simulink library "stm32f4_rtc_lib"  (R2015b)
settings: Solver=ode45  StartTime=0.0  StopTime=10.0  RelTol=1e-3
libraries: simulink x46, amg_high_precision_rtc x5
settings Model: Creator=Krisada  LastModifiedBy=Aimagin
settings DataIOCC: SaveFormat=Array  SignalLoggingSaveFormat=ModelDataLogs
settings OptimizationCC: ExpressionDepthLimit=2147483647
settings DebuggingCC: UnderspecifiedInitializationDetection=Classic  MergeDetectMultiDrivingBlocksExec=none  SolverPrmCheckMsg=warning  FcnCallInpInsideContextMsg=UseLocalSettings  StateNameClashWarn=warning  StrictBusMsg=Warning
settings HardwareCC: ProdBitPerPointer=32  ProdLargestAtomicFloat=None  ProdIntDivRoundTo=Undefined  ProdEndianess=Unspecified  ProdWordSize=32  ProdHWDeviceType=32-bit Generic
settings GRTTargetCC: CombineOutputUpdateFcns=off  GRTInterface=on
settings ConfigComp: CovModelRefEnable=Off

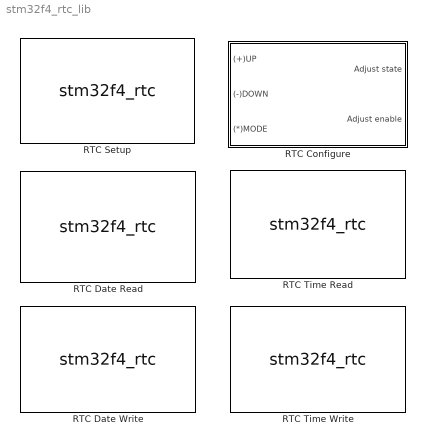
== system stm32f4_rtc_lib ==
  RTC Configure : Subsystem  mask{dummy=0}
      mask init:
      | stm32f4_rtc_configure_callback('init');
      mask Help: web(fullfile(waijungdocroot,'RTC_Configure.htm'), '-browser')
      mask Callback dummy: stm32f4_rtc_configure_callback('dummy');
      mask Display: text(0.5, 0.5, 'On-Chip RTC','ver','middle','hor','center');port_label('input', 1,'(+) UP');port_label('input', 2,'(-) DOWN');port_label('input', 3,'(*) MODE');port_label('output', 1,'State');port_label('output', 2,'Enable');
  RTC Date Read : S-Function  FunctionName=stm32f4_rtc  Parameters=inputtypearray,outputtypearray,confstr,sampletime,sampletimestr,blockid  SFunctionDeploymentMode=off  EnableBusSupport=off  mask(stm32f4_rtc){configuration=DateRead, clocksource=LSE (32.768kHz), dataformat=BIN, hourformat=HourFormat_24, inputtypearray=[0], outputtypearray=[4 3 3 3 3], confstr=["DateRead","LSE (32.768kHz)","BIN","HourFormat_24"], sampletime=-1, sampletimestr=0, blockid=stm32f4_rtc_libRTCDateRead}
      mask prompts: clocksource "Clock source"; dataformat "Format"; hourformat "Hour format"; inputtypearray "Input type array"; outputtypearray "Output type array"; confstr "Configuration string"; sampletime "Sample time (sec)"; sampletimestr "Compiled sample time (sec) in string"
      mask init:
      | stm32f4_rtc_callback('init');
      mask Help: web(fullfile(waijungdocroot,'stm32f4_rtc_read.htm'), '-browser')
      mask TypeOptions configuration: Setup | DateRead | TimeRead | DateWrite | TimeWrite
      mask Callback configuration: stm32f4_rtc_callback('configuration');
      mask TypeOptions clocksource: LSE (32.768kHz) | LSI
      mask TypeOptions dataformat: BCD | BIN
      mask Callback dataformat: stm32f4_rtc_callback('dataformat');
      mask TypeOptions hourformat: HourFormat_24 | HourFormat_12
      mask Callback confstr: stm32f4_rtc_callback('confstr');
      mask Callback sampletime: stm32f4_rtc_callback('sampletime');
      mask Callback sampletimestr: stm32f4_rtc_callback('sampletimestr');
      mask Callback blockid: stm32f4_rtc_callback('blockid');
      mask Display: text(0.05, 0.5, 'Module: RTC (DateRead)\nFormat: BIN\nTs (sec): 0','ver','middle','hor','left');port_label('output', 1,'Day');port_label('output', 2,'Date');port_label('output', 3,'Month');port_label('output', 4,'Year');
  RTC Date Write : S-Function  FunctionName=stm32f4_rtc  Parameters=inputtypearray,outputtypearray,confstr,sampletime,sampletimestr,blockid  SFunctionDeploymentMode=off  EnableBusSupport=off  mask(stm32f4_rtc){configuration=DateWrite, clocksource=LSE (32.768kHz), dataformat=BIN, hourformat=HourFormat_24, inputtypearray=[3 -1 -1 -1], outputtypearray=[0], confstr=["DateWrite","LSE (32.768kHz)","BIN","HourFormat_24"], sampletime=-1, sampletimestr=0, blockid=RTCDateWrite}
      mask prompts: clocksource "Clock source"; dataformat "Format"; hourformat "Hour format"; inputtypearray "Input type array"; outputtypearray "Output type array"; confstr "Configuration string"; sampletime "Sample time (sec)"; sampletimestr "Compiled sample time (sec) in string"
      mask init:
      | stm32f4_rtc_callback('init');
      mask Help: web(fullfile(waijungdocroot,'RTC_Date_Write.htm'), '-browser')
      mask TypeOptions configuration: Setup | DateRead | TimeRead | DateWrite | TimeWrite
      mask Callback configuration: stm32f4_rtc_callback('configuration');
      mask TypeOptions clocksource: LSE (32.768kHz) | LSI
      mask TypeOptions dataformat: BCD | BIN
      mask Callback dataformat: stm32f4_rtc_callback('dataformat');
      mask TypeOptions hourformat: HourFormat_24 | HourFormat_12
      mask Callback confstr: stm32f4_rtc_callback('confstr');
      mask Callback sampletime: stm32f4_rtc_callback('sampletime');
      mask Callback sampletimestr: stm32f4_rtc_callback('sampletimestr');
      mask Callback blockid: stm32f4_rtc_callback('blockid');
      mask Display: text(0.95, 0.5, 'Module: RTC (DateWrite)\nFormat: BIN\nTs (sec): 0','ver','middle','hor','right');port_label('input', 1,'Date');port_label('input', 2,'Month');port_label('input', 3,'Year');
  RTC Setup : S-Function  FunctionName=stm32f4_rtc  Parameters=inputtypearray,outputtypearray,confstr,sampletime,sampletimestr,blockid  SFunctionDeploymentMode=off  EnableBusSupport=off  mask(stm32f4_rtc){configuration=Setup, clocksource=LSI, dataformat=BIN, hourformat=HourFormat_24, inputtypearray=[0], outputtypearray=[0], confstr=["Setup","LSI","BIN","HourFormat_24"], sampletime=inf, sampletimestr=0, blockid=stm32f4_rtc_libRTCSetup}
      mask prompts: clocksource "Clock source"; dataformat "Format"; hourformat "Hour format"; inputtypearray "Input type array"; outputtypearray "Output type array"; confstr "Configuration string"; sampletime "Sample time (sec)"; sampletimestr "Compiled sample time (sec) in string"
      mask init:
      | stm32f4_rtc_callback('init');
      mask Help: web(fullfile(waijungdocroot,'stm32f4_rtc_setup.htm'), '-browser')
      mask TypeOptions configuration: Setup | DateRead | TimeRead | DateWrite | TimeWrite
      mask Callback configuration: stm32f4_rtc_callback('configuration');
      mask TypeOptions clocksource: LSE (32.768kHz) | LSI
      mask TypeOptions dataformat: BCD | BIN
      mask Callback dataformat: stm32f4_rtc_callback('dataformat');
      mask TypeOptions hourformat: HourFormat_24 | HourFormat_12
      mask Callback confstr: stm32f4_rtc_callback('confstr');
      mask Callback sampletime: stm32f4_rtc_callback('sampletime');
      mask Callback sampletimestr: stm32f4_rtc_callback('sampletimestr');
      mask Callback blockid: stm32f4_rtc_callback('blockid');
      mask Display: text(0.5, 0.5, 'Module: RTC (Setup)\nClock: LSI\nFormat: HourFormat_24\nTs (sec): 0','ver','middle','hor','center');
  RTC Time Read : S-Function  FunctionName=stm32f4_rtc  Parameters=inputtypearray,outputtypearray,confstr,sampletime,sampletimestr,blockid  SFunctionDeploymentMode=off  EnableBusSupport=off  mask(stm32f4_rtc){configuration=TimeRead, clocksource=LSE (32.768kHz), dataformat=BIN, hourformat=HourFormat_24, inputtypearray=[0], outputtypearray=[3 3 3 3], confstr=["TimeRead","LSE (32.768kHz)","BIN","HourFormat_24"], sampletime=-1, sampletimestr=0, blockid=stm32f4_rtc_libRTCTimeRead}
      mask prompts: clocksource "Clock source"; dataformat "Format"; hourformat "Hour format"; inputtypearray "Input type array"; outputtypearray "Output type array"; confstr "Configuration string"; sampletime "Sample time (sec)"; sampletimestr "Compiled sample time (sec) in string"
      mask init:
      | stm32f4_rtc_callback('init');
      mask Help: web(fullfile(waijungdocroot,'RTC_Time_Read.htm'), '-browser')
      mask TypeOptions configuration: Setup | DateRead | TimeRead | DateWrite | TimeWrite
      mask Callback configuration: stm32f4_rtc_callback('configuration');
      mask TypeOptions clocksource: LSE (32.768kHz) | LSI
      mask TypeOptions dataformat: BCD | BIN
      mask Callback dataformat: stm32f4_rtc_callback('dataformat');
      mask TypeOptions hourformat: HourFormat_24 | HourFormat_12
      mask Callback confstr: stm32f4_rtc_callback('confstr');
      mask Callback sampletime: stm32f4_rtc_callback('sampletime');
      mask Callback sampletimestr: stm32f4_rtc_callback('sampletimestr');
      mask Callback blockid: stm32f4_rtc_callback('blockid');
      mask Display: text(0.05, 0.5, 'Module: RTC (TimeRead)\nFormat: BIN\nTs (sec): 0','ver','middle','hor','left');port_label('output', 1,'Hour');port_label('output', 2,'Minute');port_label('output', 3,'Second');
  RTC Time Write : S-Function  FunctionName=stm32f4_rtc  Parameters=inputtypearray,outputtypearray,confstr,sampletime,sampletimestr,blockid  SFunctionDeploymentMode=off  EnableBusSupport=off  mask(stm32f4_rtc){configuration=TimeWrite, clocksource=LSE (32.768kHz), dataformat=BIN, hourformat=HourFormat_24, inputtypearray=[3 -1 -1 -1], outputtypearray=[0], confstr=["TimeWrite","LSE (32.768kHz)","BIN","HourFormat_24"], sampletime=-1, sampletimestr=0, blockid=stm32f4_rtc_libRTCTimeWrite}
      mask prompts: clocksource "Clock source"; dataformat "Format"; hourformat "Hour format"; inputtypearray "Input type array"; outputtypearray "Output type array"; confstr "Configuration string"; sampletime "Sample time (sec)"; sampletimestr "Compiled sample time (sec) in string"
      mask init:
      | stm32f4_rtc_callback('init');
      mask Help: web(fullfile(waijungdocroot,'RTC_Time_Write.htm'), '-browser')
      mask TypeOptions configuration: Setup | DateRead | TimeRead | DateWrite | TimeWrite
      mask Callback configuration: stm32f4_rtc_callback('configuration');
      mask TypeOptions clocksource: LSE (32.768kHz) | LSI
      mask TypeOptions dataformat: BCD | BIN
      mask Callback dataformat: stm32f4_rtc_callback('dataformat');
      mask TypeOptions hourformat: HourFormat_24 | HourFormat_12
      mask Callback confstr: stm32f4_rtc_callback('confstr');
      mask Callback sampletime: stm32f4_rtc_callback('sampletime');
      mask Callback sampletimestr: stm32f4_rtc_callback('sampletimestr');
      mask Callback blockid: stm32f4_rtc_callback('blockid');
      mask Display: text(0.95, 0.5, 'Module: RTC (TimeWrite)\nFormat: BIN\nTs (sec): 0','ver','middle','hor','right');port_label('input', 1,'Hour');port_label('input', 2,'Minute');port_label('input', 3,'Second');

== system stm32f4_rtc_lib/RTC Configure ==
  (+)UP : Inport
  (-)DOWN : Inport  Port=2
  (*)MODE : Inport  Port=3
  Debouce4 : Subsystem  TreatAsAtomicUnit=on  mask{mode=Toggle Latch, prescale=256, debouce=255}
      mask prompts: prescale "Prescale (Debouce count)"; debouce "Debouce value"
      settings: RTWFcnNameOpts=Use subsystem name  RTWFileNameOpts=Use function name
      mask TypeOptions mode: Normal | Single Pulse | Toggle Latch
      mask Callback mode: waijung_intput_validation_callback('mode');
      mask TypeOptions prescale: 4 | 8 | 16 | 32 | 64 | 128 | 256 | 512 | 1024 | 2048 | 4096 | 8192
      mask Callback debouce: waijung_intput_validation_callback('prescale');
      mask Display: disp('Button Pressed\n(Toggle Latch)\nDebouce count: 256');
  Enabled Subsystem : Subsystem  TreatAsAtomicUnit=on
  Adjust state : Outport
  Adjust enable : Outport  Port=2
  wires:
  (+)UP/1 -> Enabled Subsystem/1(UP)
  (-)DOWN/1 -> Enabled Subsystem/2(DOWN)
  (*)MODE/1 -> Debouce4/1(In1), Enabled Subsystem/3(MODE)
  Debouce4/1(Out1) -> Enabled Subsystem/Enable, Adjust enable/1
  Enabled Subsystem/1(Adjust state) -> Adjust state/1

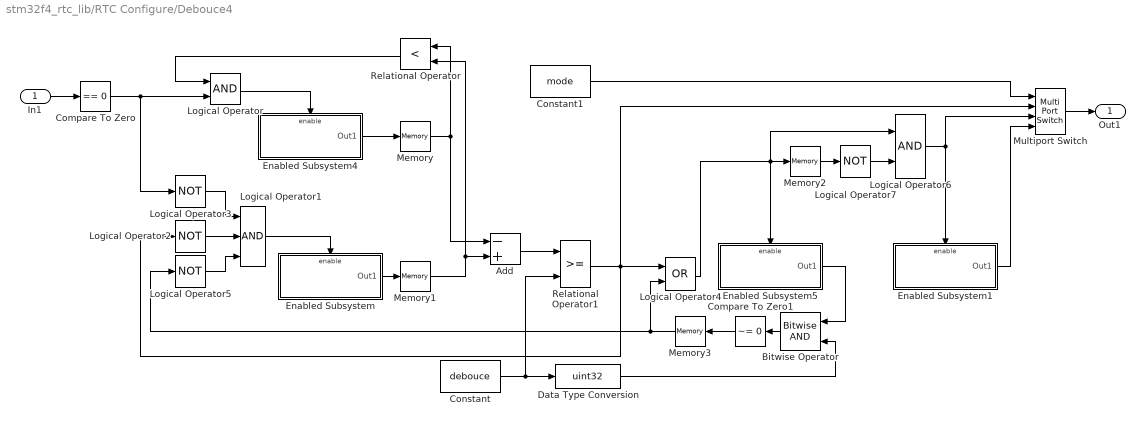
== system stm32f4_rtc_lib/RTC Configure/Debouce4 ==
  In1 : Inport
  Add : Sum  Inputs=-+  OutDataTypeStr=int32
  Bitwise Operator : simulink/Logic and Bit Operations/Bitwise Operator  logicop=AND  UseBitMask=off  NumInputPorts=2  BitMask=debouce  BitMaskRealWorld=Stored Integer
  Compare To Zero : simulink/Logic and Bit Operations/Compare To Zero  SystemSampleTime=-1  relop===  LogicOutDataTypeMode=uint8  ZeroCross=off
  Compare To Zero1 : simulink/Logic and Bit Operations/Compare To Zero  SystemSampleTime=-1  relop=~=  LogicOutDataTypeMode=boolean  ZeroCross=off
  Constant : Constant  Value=debouce  OutDataTypeStr=int32
  Constant1 : Constant  Value=mode  OutDataTypeStr=int32
  Data Type Conversion : DataTypeConversion  OutDataTypeStr=uint32
  Enabled Subsystem : Subsystem  TreatAsAtomicUnit=on
  Enabled Subsystem1 : Subsystem  TreatAsAtomicUnit=on
  Enabled Subsystem4 : Subsystem  TreatAsAtomicUnit=on
  Enabled Subsystem5 : Subsystem  TreatAsAtomicUnit=on
  Logical Operator : Logic  AllPortsSameDT=off  OutDataTypeStr=boolean
  Logical Operator1 : Logic  Inputs=3  AllPortsSameDT=off  OutDataTypeStr=boolean
  Logical Operator{2..3,5,7} (4 alike) : Logic  Operator=NOT  AllPortsSameDT=off  OutDataTypeStr=boolean
  Logical Operator4 : Logic  Operator=OR  AllPortsSameDT=off  OutDataTypeStr=boolean
  Logical Operator6 : Logic  AllPortsSameDT=off  OutDataTypeStr=boolean
  Memory{,1..3} (4 alike) : Memory  LinearizeMemory=on
  Multiport Switch : MultiPortSwitch
  Relational Operator : RelationalOperator  Operator=<  OutDataTypeStr=boolean
  Relational Operator1 : RelationalOperator  OutDataTypeStr=boolean  InputSameDT=on
  Out1 : Outport
  wires:
  Constant1/1 -> Multiport Switch/1
  Multiport Switch/1 -> Out1/1
  Data Type Conversion/1 -> Bitwise Operator/2
  Enabled Subsystem1/1(Out1) -> Multiport Switch/4
  Logical Operator6/1 -> Enabled Subsystem1/Enable, Multiport Switch/3
  In1/1 -> Compare To Zero/1
  Enabled Subsystem/1(Out1) -> Memory1/1
  Enabled Subsystem4/1(Out1) -> Memory/1
  Memory/1 -> Relational Operator/1, Add/1
  Memory1/1 -> Add/2, Relational Operator/2
  Compare To Zero/1 -> Logical Operator/2, Logical Operator3/1
  Logical Operator/1 -> Enabled Subsystem4/Enable
  Relational Operator/1 -> Logical Operator/1
  Add/1 -> Relational Operator1/1
  Constant/1 -> Data Type Conversion/1, Relational Operator1/2
  Logical Operator2/1 -> Logical Operator1/2
  Memory3/1 -> Logical Operator4/2, Logical Operator5/1
  Logical Operator5/1 -> Logical Operator1/3
  Logical Operator3/1 -> Logical Operator1/1
  Compare To Zero1/1 -> Memory3/1
  Bitwise Operator/1 -> Compare To Zero1/1
  Enabled Subsystem5/1(Out1) -> Bitwise Operator/1
  Logical Operator4/1 -> Enabled Subsystem5/Enable, Memory2/1, Logical Operator6/1
  Memory2/1 -> Logical Operator7/1
  Logical Operator7/1 -> Logical Operator6/2
  Relational Operator1/1 -> Multiport Switch/2, Logical Operator4/1, Logical Operator2/1
  Logical Operator1/1 -> Enabled Subsystem/Enable

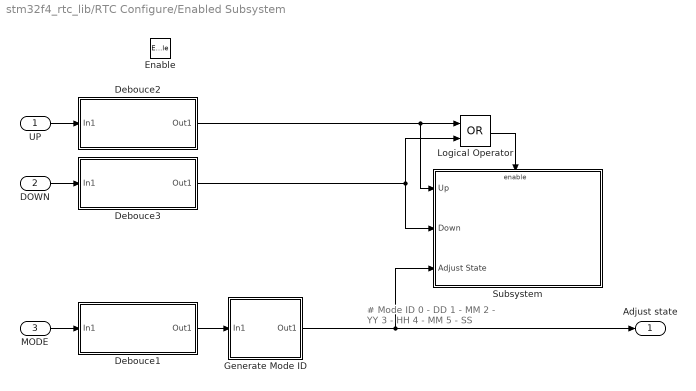
== system stm32f4_rtc_lib/RTC Configure/Enabled Subsystem ==
  note: # Mode ID
      | 0 - DD
      | 1 - MM
      | 2 - YY
      | 3 - HH
      | 4 - MM
      | 5 - SS
  UP : Inport
  DOWN : Inport  Port=2
  MODE : Inport  Port=3
  Enable : EnablePort  PropagateVarSize=During execution
  Debouce1 : Subsystem  TreatAsAtomicUnit=on  mask{mode=Single Pulse, prescale=4, debouce=7}
      mask prompts: prescale "Prescale (Debouce count)"; debouce "Debouce value"
      settings: RTWFcnNameOpts=Use subsystem name  RTWFileNameOpts=Use function name
      mask TypeOptions mode: Normal | Single Pulse | Toggle Latch
      mask Callback mode: waijung_intput_validation_callback('mode');
      mask TypeOptions prescale: 4 | 8 | 16 | 32 | 64 | 128 | 256 | 512 | 1024 | 2048 | 4096 | 8192
      mask Callback debouce: waijung_intput_validation_callback('prescale');
      mask Display: disp('Button Pressed\n(Normal)');
  Debouce2 : Subsystem  TreatAsAtomicUnit=on  mask{mode=Single Pulse, prescale=4, debouce=3}
      mask prompts: prescale "Prescale (Debouce count)"; debouce "Debouce value"
      settings: RTWFcnNameOpts=Use subsystem name  RTWFileNameOpts=Use function name
      mask TypeOptions mode: Normal | Single Pulse | Toggle Latch
      mask Callback mode: waijung_intput_validation_callback('mode');
      mask TypeOptions prescale: 4 | 8 | 16 | 32 | 64 | 128 | 256 | 512 | 1024 | 2048 | 4096 | 8192
      mask Callback debouce: waijung_intput_validation_callback('prescale');
      mask Display: disp('Button Pressed\n(Normal)');
  Debouce3 : Subsystem  TreatAsAtomicUnit=on  mask{mode=Single Pulse, prescale=4, debouce=3}
      mask prompts: prescale "Prescale (Debouce count)"; debouce "Debouce value"
      settings: RTWFcnNameOpts=Use subsystem name  RTWFileNameOpts=Use function name
      mask TypeOptions mode: Normal | Single Pulse | Toggle Latch
      mask Callback mode: waijung_intput_validation_callback('mode');
      mask TypeOptions prescale: 4 | 8 | 16 | 32 | 64 | 128 | 256 | 512 | 1024 | 2048 | 4096 | 8192
      mask Callback debouce: waijung_intput_validation_callback('prescale');
      mask Display: disp('Button Pressed\n(Normal)');
  Generate Mode ID : Subsystem
  Logical Operator : Logic  Operator=OR  AllPortsSameDT=off  OutDataTypeStr=boolean
  Subsystem : Subsystem
  Adjust state : Outport
  wires:
  UP/1 -> Debouce2/1(In1)
  DOWN/1 -> Debouce3/1(In1)
  MODE/1 -> Debouce1/1(In1)
  Debouce1/1(Out1) -> Generate Mode ID/1(In1)
  Generate Mode ID/1(Out1) -> Adjust state/1, Subsystem/3(Adjust State)
  Debouce3/1(Out1) -> Logical Operator/2, Subsystem/2(Down)
  Debouce2/1(Out1) -> Logical Operator/1, Subsystem/1(Up)
  Logical Operator/1 -> Subsystem/Enable

== system stm32f4_rtc_lib/RTC Configure/Debouce4/Enabled Subsystem ==
  Enable : EnablePort  PropagateVarSize=During execution
  Counter Free-Running : simulink/Sources/Counter Free-Running  SystemSampleTime=-1  NumBits=32  tsamp=-1
  Out1 : Outport  InitialOutput=0
  wires:
  Counter Free-Running/1 -> Out1/1

== system stm32f4_rtc_lib/RTC Configure/Debouce4/Enabled Subsystem1 ==
  Enable : EnablePort  PropagateVarSize=During execution
  Bitwise Operator : simulink/Logic and Bit Operations/Bitwise Operator  logicop=AND  UseBitMask=on  BitMask=1  BitMaskRealWorld=Stored Integer
  Compare To Zero : simulink/Logic and Bit Operations/Compare To Zero  SystemSampleTime=-1  relop===  LogicOutDataTypeMode=uint8  ZeroCross=off
  Counter Free-Running : simulink/Sources/Counter Free-Running  SystemSampleTime=-1  NumBits=32  tsamp=-1
  Out1 : Outport  InitialOutput=0
  wires:
  Counter Free-Running/1 -> Bitwise Operator/1
  Bitwise Operator/1 -> Compare To Zero/1
  Compare To Zero/1 -> Out1/1

== system stm32f4_rtc_lib/RTC Configure/Debouce4/Enabled Subsystem4 ==
  Enable : EnablePort  PropagateVarSize=During execution
  Counter Free-Running : simulink/Sources/Counter Free-Running  SystemSampleTime=-1  NumBits=32  tsamp=-1
  Out1 : Outport  InitialOutput=0
  wires:
  Counter Free-Running/1 -> Out1/1

== system stm32f4_rtc_lib/RTC Configure/Debouce4/Enabled Subsystem5 ==
  Enable : EnablePort  PropagateVarSize=During execution
  Counter Free-Running : simulink/Sources/Counter Free-Running  SystemSampleTime=-1  NumBits=32  tsamp=-1
  Out1 : Outport  InitialOutput=0
  wires:
  Counter Free-Running/1 -> Out1/1

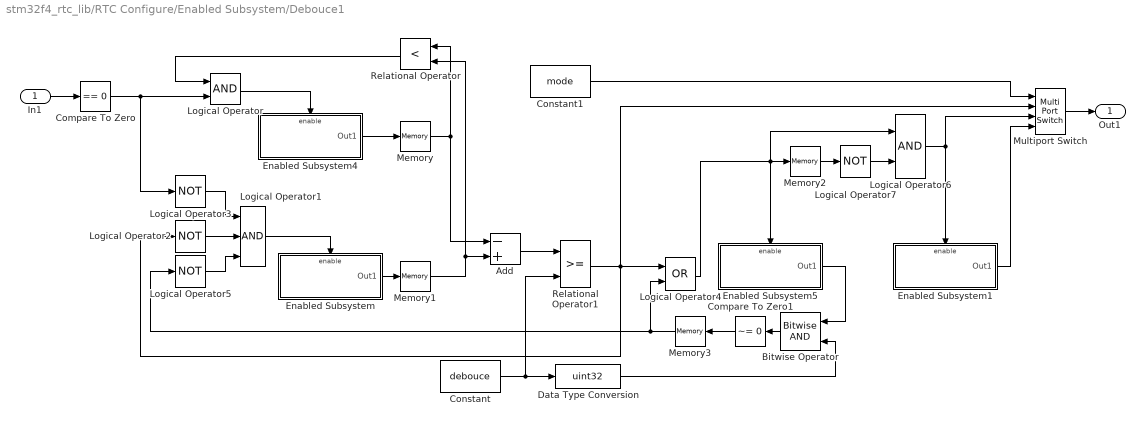
== system stm32f4_rtc_lib/RTC Configure/Enabled Subsystem/Debouce1 ==
  In1 : Inport
  Add : Sum  Inputs=-+  OutDataTypeStr=int32
  Bitwise Operator : simulink/Logic and Bit Operations/Bitwise Operator  logicop=AND  UseBitMask=off  NumInputPorts=2  BitMask=debouce  BitMaskRealWorld=Stored Integer
  Compare To Zero : simulink/Logic and Bit Operations/Compare To Zero  SystemSampleTime=-1  relop===  LogicOutDataTypeMode=uint8  ZeroCross=off
  Compare To Zero1 : simulink/Logic and Bit Operations/Compare To Zero  SystemSampleTime=-1  relop=~=  LogicOutDataTypeMode=boolean  ZeroCross=off
  Constant : Constant  Value=debouce  OutDataTypeStr=int32
  Constant1 : Constant  Value=mode  OutDataTypeStr=int32
  Data Type Conversion : DataTypeConversion  OutDataTypeStr=uint32
  Enabled Subsystem : Subsystem  TreatAsAtomicUnit=on
  Enabled Subsystem1 : Subsystem  TreatAsAtomicUnit=on
  Enabled Subsystem4 : Subsystem  TreatAsAtomicUnit=on
  Enabled Subsystem5 : Subsystem  TreatAsAtomicUnit=on
  Logical Operator : Logic  AllPortsSameDT=off  OutDataTypeStr=boolean
  Logical Operator1 : Logic  Inputs=3  AllPortsSameDT=off  OutDataTypeStr=boolean
  Logical Operator{2..3,5,7} (4 alike) : Logic  Operator=NOT  AllPortsSameDT=off  OutDataTypeStr=boolean
  Logical Operator4 : Logic  Operator=OR  AllPortsSameDT=off  OutDataTypeStr=boolean
  Logical Operator6 : Logic  AllPortsSameDT=off  OutDataTypeStr=boolean
  Memory{,1..3} (4 alike) : Memory  LinearizeMemory=on
  Multiport Switch : MultiPortSwitch
  Relational Operator : RelationalOperator  Operator=<  OutDataTypeStr=boolean
  Relational Operator1 : RelationalOperator  OutDataTypeStr=boolean  InputSameDT=on
  Out1 : Outport
  wires:
  Constant1/1 -> Multiport Switch/1
  Multiport Switch/1 -> Out1/1
  Data Type Conversion/1 -> Bitwise Operator/2
  Enabled Subsystem1/1(Out1) -> Multiport Switch/4
  Logical Operator6/1 -> Enabled Subsystem1/Enable, Multiport Switch/3
  In1/1 -> Compare To Zero/1
  Enabled Subsystem/1(Out1) -> Memory1/1
  Enabled Subsystem4/1(Out1) -> Memory/1
  Memory/1 -> Relational Operator/1, Add/1
  Memory1/1 -> Add/2, Relational Operator/2
  Compare To Zero/1 -> Logical Operator/2, Logical Operator3/1
  Logical Operator/1 -> Enabled Subsystem4/Enable
  Relational Operator/1 -> Logical Operator/1
  Add/1 -> Relational Operator1/1
  Constant/1 -> Data Type Conversion/1, Relational Operator1/2
  Logical Operator2/1 -> Logical Operator1/2
  Memory3/1 -> Logical Operator4/2, Logical Operator5/1
  Logical Operator5/1 -> Logical Operator1/3
  Logical Operator3/1 -> Logical Operator1/1
  Compare To Zero1/1 -> Memory3/1
  Bitwise Operator/1 -> Compare To Zero1/1
  Enabled Subsystem5/1(Out1) -> Bitwise Operator/1
  Logical Operator4/1 -> Enabled Subsystem5/Enable, Memory2/1, Logical Operator6/1
  Memory2/1 -> Logical Operator7/1
  Logical Operator7/1 -> Logical Operator6/2
  Relational Operator1/1 -> Multiport Switch/2, Logical Operator4/1, Logical Operator2/1
  Logical Operator1/1 -> Enabled Subsystem/Enable

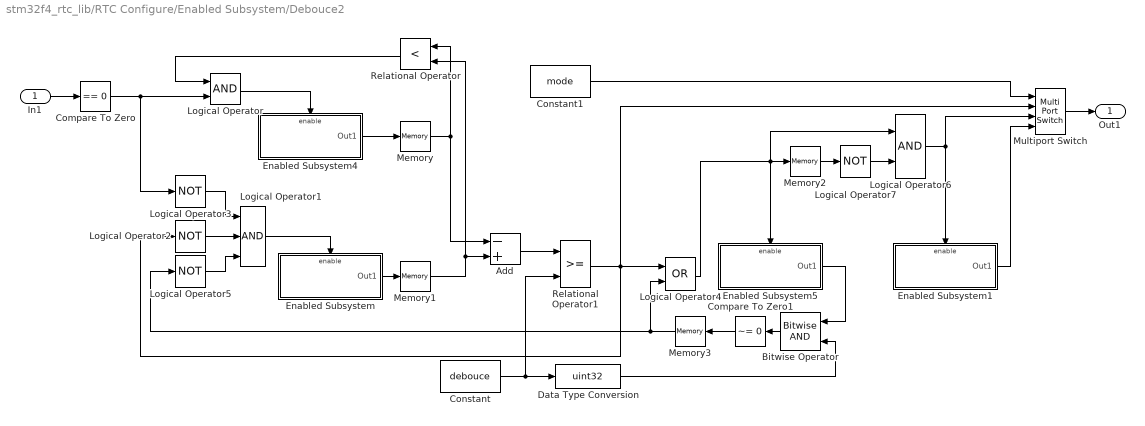
== system stm32f4_rtc_lib/RTC Configure/Enabled Subsystem/Debouce2 ==
  In1 : Inport
  Add : Sum  Inputs=-+  OutDataTypeStr=int32
  Bitwise Operator : simulink/Logic and Bit Operations/Bitwise Operator  logicop=AND  UseBitMask=off  NumInputPorts=2  BitMask=debouce  BitMaskRealWorld=Stored Integer
  Compare To Zero : simulink/Logic and Bit Operations/Compare To Zero  SystemSampleTime=-1  relop===  LogicOutDataTypeMode=uint8  ZeroCross=off
  Compare To Zero1 : simulink/Logic and Bit Operations/Compare To Zero  SystemSampleTime=-1  relop=~=  LogicOutDataTypeMode=boolean  ZeroCross=off
  Constant : Constant  Value=debouce  OutDataTypeStr=int32
  Constant1 : Constant  Value=mode  OutDataTypeStr=int32
  Data Type Conversion : DataTypeConversion  OutDataTypeStr=uint32
  Enabled Subsystem : Subsystem  TreatAsAtomicUnit=on
  Enabled Subsystem1 : Subsystem  TreatAsAtomicUnit=on
  Enabled Subsystem4 : Subsystem  TreatAsAtomicUnit=on
  Enabled Subsystem5 : Subsystem  TreatAsAtomicUnit=on
  Logical Operator : Logic  AllPortsSameDT=off  OutDataTypeStr=boolean
  Logical Operator1 : Logic  Inputs=3  AllPortsSameDT=off  OutDataTypeStr=boolean
  Logical Operator{2..3,5,7} (4 alike) : Logic  Operator=NOT  AllPortsSameDT=off  OutDataTypeStr=boolean
  Logical Operator4 : Logic  Operator=OR  AllPortsSameDT=off  OutDataTypeStr=boolean
  Logical Operator6 : Logic  AllPortsSameDT=off  OutDataTypeStr=boolean
  Memory{,1..3} (4 alike) : Memory  LinearizeMemory=on
  Multiport Switch : MultiPortSwitch
  Relational Operator : RelationalOperator  Operator=<  OutDataTypeStr=boolean
  Relational Operator1 : RelationalOperator  OutDataTypeStr=boolean  InputSameDT=on
  Out1 : Outport
  wires:
  Constant1/1 -> Multiport Switch/1
  Multiport Switch/1 -> Out1/1
  Data Type Conversion/1 -> Bitwise Operator/2
  Enabled Subsystem1/1(Out1) -> Multiport Switch/4
  Logical Operator6/1 -> Enabled Subsystem1/Enable, Multiport Switch/3
  In1/1 -> Compare To Zero/1
  Enabled Subsystem/1(Out1) -> Memory1/1
  Enabled Subsystem4/1(Out1) -> Memory/1
  Memory/1 -> Relational Operator/1, Add/1
  Memory1/1 -> Add/2, Relational Operator/2
  Compare To Zero/1 -> Logical Operator/2, Logical Operator3/1
  Logical Operator/1 -> Enabled Subsystem4/Enable
  Relational Operator/1 -> Logical Operator/1
  Add/1 -> Relational Operator1/1
  Constant/1 -> Data Type Conversion/1, Relational Operator1/2
  Logical Operator2/1 -> Logical Operator1/2
  Memory3/1 -> Logical Operator4/2, Logical Operator5/1
  Logical Operator5/1 -> Logical Operator1/3
  Logical Operator3/1 -> Logical Operator1/1
  Compare To Zero1/1 -> Memory3/1
  Bitwise Operator/1 -> Compare To Zero1/1
  Enabled Subsystem5/1(Out1) -> Bitwise Operator/1
  Logical Operator4/1 -> Enabled Subsystem5/Enable, Memory2/1, Logical Operator6/1
  Memory2/1 -> Logical Operator7/1
  Logical Operator7/1 -> Logical Operator6/2
  Relational Operator1/1 -> Multiport Switch/2, Logical Operator4/1, Logical Operator2/1
  Logical Operator1/1 -> Enabled Subsystem/Enable

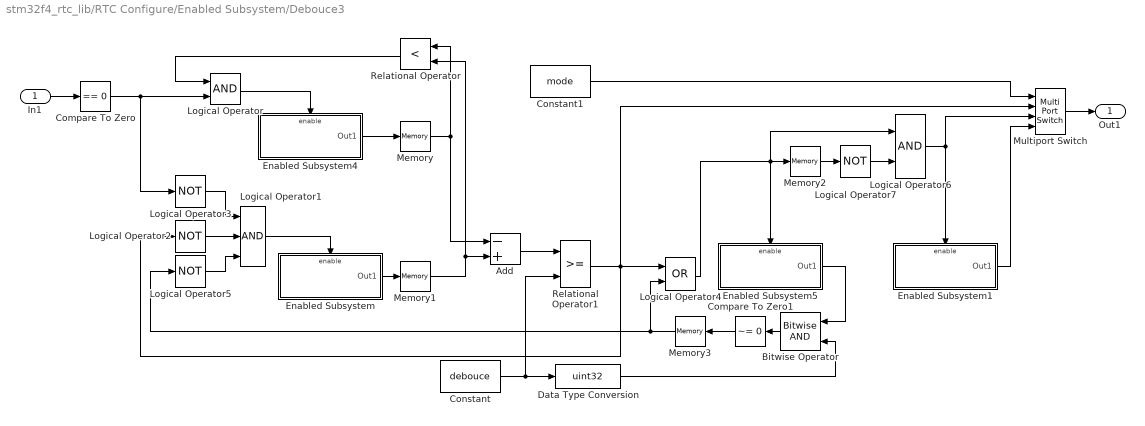
== system stm32f4_rtc_lib/RTC Configure/Enabled Subsystem/Debouce3 ==
  In1 : Inport
  Add : Sum  Inputs=-+  OutDataTypeStr=int32
  Bitwise Operator : simulink/Logic and Bit Operations/Bitwise Operator  logicop=AND  UseBitMask=off  NumInputPorts=2  BitMask=debouce  BitMaskRealWorld=Stored Integer
  Compare To Zero : simulink/Logic and Bit Operations/Compare To Zero  SystemSampleTime=-1  relop===  LogicOutDataTypeMode=uint8  ZeroCross=off
  Compare To Zero1 : simulink/Logic and Bit Operations/Compare To Zero  SystemSampleTime=-1  relop=~=  LogicOutDataTypeMode=boolean  ZeroCross=off
  Constant : Constant  Value=debouce  OutDataTypeStr=int32
  Constant1 : Constant  Value=mode  OutDataTypeStr=int32
  Data Type Conversion : DataTypeConversion  OutDataTypeStr=uint32
  Enabled Subsystem : Subsystem  TreatAsAtomicUnit=on
  Enabled Subsystem1 : Subsystem  TreatAsAtomicUnit=on
  Enabled Subsystem4 : Subsystem  TreatAsAtomicUnit=on
  Enabled Subsystem5 : Subsystem  TreatAsAtomicUnit=on
  Logical Operator : Logic  AllPortsSameDT=off  OutDataTypeStr=boolean
  Logical Operator1 : Logic  Inputs=3  AllPortsSameDT=off  OutDataTypeStr=boolean
  Logical Operator{2..3,5,7} (4 alike) : Logic  Operator=NOT  AllPortsSameDT=off  OutDataTypeStr=boolean
  Logical Operator4 : Logic  Operator=OR  AllPortsSameDT=off  OutDataTypeStr=boolean
  Logical Operator6 : Logic  AllPortsSameDT=off  OutDataTypeStr=boolean
  Memory{,1..3} (4 alike) : Memory  LinearizeMemory=on
  Multiport Switch : MultiPortSwitch
  Relational Operator : RelationalOperator  Operator=<  OutDataTypeStr=boolean
  Relational Operator1 : RelationalOperator  OutDataTypeStr=boolean  InputSameDT=on
  Out1 : Outport
  wires:
  Constant1/1 -> Multiport Switch/1
  Multiport Switch/1 -> Out1/1
  Data Type Conversion/1 -> Bitwise Operator/2
  Enabled Subsystem1/1(Out1) -> Multiport Switch/4
  Logical Operator6/1 -> Enabled Subsystem1/Enable, Multiport Switch/3
  In1/1 -> Compare To Zero/1
  Enabled Subsystem/1(Out1) -> Memory1/1
  Enabled Subsystem4/1(Out1) -> Memory/1
  Memory/1 -> Relational Operator/1, Add/1
  Memory1/1 -> Add/2, Relational Operator/2
  Compare To Zero/1 -> Logical Operator/2, Logical Operator3/1
  Logical Operator/1 -> Enabled Subsystem4/Enable
  Relational Operator/1 -> Logical Operator/1
  Add/1 -> Relational Operator1/1
  Constant/1 -> Data Type Conversion/1, Relational Operator1/2
  Logical Operator2/1 -> Logical Operator1/2
  Memory3/1 -> Logical Operator4/2, Logical Operator5/1
  Logical Operator5/1 -> Logical Operator1/3
  Logical Operator3/1 -> Logical Operator1/1
  Compare To Zero1/1 -> Memory3/1
  Bitwise Operator/1 -> Compare To Zero1/1
  Enabled Subsystem5/1(Out1) -> Bitwise Operator/1
  Logical Operator4/1 -> Enabled Subsystem5/Enable, Memory2/1, Logical Operator6/1
  Memory2/1 -> Logical Operator7/1
  Logical Operator7/1 -> Logical Operator6/2
  Relational Operator1/1 -> Multiport Switch/2, Logical Operator4/1, Logical Operator2/1
  Logical Operator1/1 -> Enabled Subsystem/Enable

== system stm32f4_rtc_lib/RTC Configure/Enabled Subsystem/Generate Mode ID ==
  note: # check unused state
  In1 : Inport
  Compare To Constant : simulink/Logic and Bit Operations/Compare To Constant  SystemSampleTime=-1  relop=>  const=5  LogicOutDataTypeMode=boolean  ZeroCross=off
  Enabled Subsystem2 : Subsystem  TreatAsAtomicUnit=on
  Logical Operator : Logic  Operator=OR  AllPortsSameDT=off  OutDataTypeStr=boolean
  Unit Delay : UnitDelay  SampleTime=-1
  Out1 : Outport
  wires:
  Enabled Subsystem2/1(Out1) -> Unit Delay/1, Out1/1
  Logical Operator/1 -> Enabled Subsystem2/Enable
  Compare To Constant/1 -> Logical Operator/1
  Unit Delay/1 -> Compare To Constant/1
  In1/1 -> Logical Operator/2

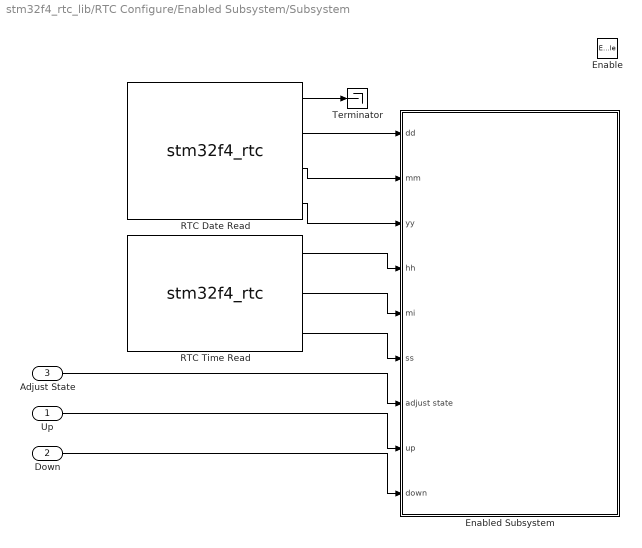
== system stm32f4_rtc_lib/RTC Configure/Enabled Subsystem/Subsystem ==
  Up : Inport
  Down : Inport  Port=2
  Adjust State : Inport  Port=3
  Enable : EnablePort  PropagateVarSize=During execution
  Enabled Subsystem : Subsystem  TreatAsAtomicUnit=on
  RTC Date Read : S-Function  FunctionName=stm32f4_rtc  Parameters=inputtypearray,outputtypearray,confstr,sampletime,sampletimestr,blockid  SFunctionDeploymentMode=off  EnableBusSupport=off  mask(stm32f4_rtc){configuration=DateRead, clocksource=LSE (32.768kHz), dataformat=BIN, hourformat=HourFormat_24, inputtypearray=[0], outputtypearray=[4 3 3 3 3], confstr=["DateRead","LSE (32.768kHz)","BIN","HourFormat_24"], sampletime=0.01, sampletimestr=0, blockid=stm32f4_rtc_libRTCConfigureEnabledSubsystemSubsystemRTCDateRead}
      mask prompts: clocksource "Clock source"; dataformat "Format"; hourformat "Hour format"; inputtypearray "Input type array"; outputtypearray "Output type array"; confstr "Configuration string"; sampletime "Sample time (sec)"; sampletimestr "Compiled sample time (sec) in string"
      mask init:
      | stm32f4_rtc_callback('init');
      mask Help: web(fullfile(waijungdocroot,'stm32f4_rtc_setup.htm'), '-browser')
      mask TypeOptions configuration: Setup | DateRead | TimeRead | DateWrite | TimeWrite
      mask Callback configuration: stm32f4_rtc_callback('configuration');
      mask TypeOptions clocksource: LSE (32.768kHz) | LSI
      mask TypeOptions dataformat: BCD | BIN
      mask Callback dataformat: stm32f4_rtc_callback('dataformat');
      mask TypeOptions hourformat: HourFormat_24 | HourFormat_12
      mask Callback confstr: stm32f4_rtc_callback('confstr');
      mask Callback sampletime: stm32f4_rtc_callback('sampletime');
      mask Callback sampletimestr: stm32f4_rtc_callback('sampletimestr');
      mask Callback blockid: stm32f4_rtc_callback('blockid');
      mask Display: text(0.05, 0.5, 'Module: RTC (DateRead)\nFormat: BIN\nTs (sec): 0','ver','middle','hor','left');port_label('output', 1,'Day');port_label('output', 2,'Date');port_label('output', 3,'Month');port_label('output', 4,'Year');
  RTC Time Read : S-Function  FunctionName=stm32f4_rtc  Parameters=inputtypearray,outputtypearray,confstr,sampletime,sampletimestr,blockid  SFunctionDeploymentMode=off  EnableBusSupport=off  mask(stm32f4_rtc){configuration=TimeRead, clocksource=LSE (32.768kHz), dataformat=BIN, hourformat=HourFormat_24, inputtypearray=[0], outputtypearray=[3 3 3 3], confstr=["TimeRead","LSE (32.768kHz)","BIN","HourFormat_24"], sampletime=0.01, sampletimestr=0, blockid=stm32f4_rtc_libRTCConfigureEnabledSubsystemSubsystemRTCTimeRead}
      mask prompts: clocksource "Clock source"; dataformat "Format"; hourformat "Hour format"; inputtypearray "Input type array"; outputtypearray "Output type array"; confstr "Configuration string"; sampletime "Sample time (sec)"; sampletimestr "Compiled sample time (sec) in string"
      mask init:
      | stm32f4_rtc_callback('init');
      mask Help: web(fullfile(waijungdocroot,'stm32f4_rtc_setup.htm'), '-browser')
      mask TypeOptions configuration: Setup | DateRead | TimeRead | DateWrite | TimeWrite
      mask Callback configuration: stm32f4_rtc_callback('configuration');
      mask TypeOptions clocksource: LSE (32.768kHz) | LSI
      mask TypeOptions dataformat: BCD | BIN
      mask Callback dataformat: stm32f4_rtc_callback('dataformat');
      mask TypeOptions hourformat: HourFormat_24 | HourFormat_12
      mask Callback confstr: stm32f4_rtc_callback('confstr');
      mask Callback sampletime: stm32f4_rtc_callback('sampletime');
      mask Callback sampletimestr: stm32f4_rtc_callback('sampletimestr');
      mask Callback blockid: stm32f4_rtc_callback('blockid');
      mask Display: text(0.05, 0.5, 'Module: RTC (TimeRead)\nFormat: BIN\nTs (sec): 0','ver','middle','hor','left');port_label('output', 1,'Hour');port_label('output', 2,'Minute');port_label('output', 3,'Second');
  Terminator : Terminator
  wires:
  RTC Date Read/3 -> Enabled Subsystem/2(mm)
  RTC Date Read/4 -> Enabled Subsystem/3(yy)
  RTC Date Read/1 -> Terminator/1
  Adjust State/1 -> Enabled Subsystem/7(adjust state)
  Up/1 -> Enabled Subsystem/8(up)
  Down/1 -> Enabled Subsystem/9(down)
  RTC Time Read/1 -> Enabled Subsystem/4(hh)
  RTC Time Read/2 -> Enabled Subsystem/5(mi)
  RTC Time Read/3 -> Enabled Subsystem/6(ss)
  RTC Date Read/2 -> Enabled Subsystem/1(dd)

== system stm32f4_rtc_lib/RTC Configure/Enabled Subsystem/Debouce1/Enabled Subsystem ==
  Enable : EnablePort  PropagateVarSize=During execution
  Counter Free-Running : simulink/Sources/Counter Free-Running  SystemSampleTime=-1  NumBits=32  tsamp=-1
  Out1 : Outport  InitialOutput=0
  wires:
  Counter Free-Running/1 -> Out1/1

== system stm32f4_rtc_lib/RTC Configure/Enabled Subsystem/Debouce1/Enabled Subsystem1 ==
  Enable : EnablePort  PropagateVarSize=During execution
  Bitwise Operator : simulink/Logic and Bit Operations/Bitwise Operator  logicop=AND  UseBitMask=on  BitMask=1  BitMaskRealWorld=Stored Integer
  Compare To Zero : simulink/Logic and Bit Operations/Compare To Zero  SystemSampleTime=-1  relop===  LogicOutDataTypeMode=uint8  ZeroCross=off
  Counter Free-Running : simulink/Sources/Counter Free-Running  SystemSampleTime=-1  NumBits=32  tsamp=-1
  Out1 : Outport  InitialOutput=0
  wires:
  Counter Free-Running/1 -> Bitwise Operator/1
  Bitwise Operator/1 -> Compare To Zero/1
  Compare To Zero/1 -> Out1/1

== system stm32f4_rtc_lib/RTC Configure/Enabled Subsystem/Debouce1/Enabled Subsystem4 ==
  Enable : EnablePort  PropagateVarSize=During execution
  Counter Free-Running : simulink/Sources/Counter Free-Running  SystemSampleTime=-1  NumBits=32  tsamp=-1
  Out1 : Outport  InitialOutput=0
  wires:
  Counter Free-Running/1 -> Out1/1

== system stm32f4_rtc_lib/RTC Configure/Enabled Subsystem/Debouce1/Enabled Subsystem5 ==
  Enable : EnablePort  PropagateVarSize=During execution
  Counter Free-Running : simulink/Sources/Counter Free-Running  SystemSampleTime=-1  NumBits=32  tsamp=-1
  Out1 : Outport  InitialOutput=0
  wires:
  Counter Free-Running/1 -> Out1/1

== system stm32f4_rtc_lib/RTC Configure/Enabled Subsystem/Debouce2/Enabled Subsystem ==
  Enable : EnablePort  PropagateVarSize=During execution
  Counter Free-Running : simulink/Sources/Counter Free-Running  SystemSampleTime=-1  NumBits=32  tsamp=-1
  Out1 : Outport  InitialOutput=0
  wires:
  Counter Free-Running/1 -> Out1/1

== system stm32f4_rtc_lib/RTC Configure/Enabled Subsystem/Debouce2/Enabled Subsystem1 ==
  Enable : EnablePort  PropagateVarSize=During execution
  Bitwise Operator : simulink/Logic and Bit Operations/Bitwise Operator  logicop=AND  UseBitMask=on  BitMask=1  BitMaskRealWorld=Stored Integer
  Compare To Zero : simulink/Logic and Bit Operations/Compare To Zero  SystemSampleTime=-1  relop===  LogicOutDataTypeMode=uint8  ZeroCross=off
  Counter Free-Running : simulink/Sources/Counter Free-Running  SystemSampleTime=-1  NumBits=32  tsamp=-1
  Out1 : Outport  InitialOutput=0
  wires:
  Counter Free-Running/1 -> Bitwise Operator/1
  Bitwise Operator/1 -> Compare To Zero/1
  Compare To Zero/1 -> Out1/1

== system stm32f4_rtc_lib/RTC Configure/Enabled Subsystem/Debouce2/Enabled Subsystem4 ==
  Enable : EnablePort  PropagateVarSize=During execution
  Counter Free-Running : simulink/Sources/Counter Free-Running  SystemSampleTime=-1  NumBits=32  tsamp=-1
  Out1 : Outport  InitialOutput=0
  wires:
  Counter Free-Running/1 -> Out1/1

== system stm32f4_rtc_lib/RTC Configure/Enabled Subsystem/Debouce2/Enabled Subsystem5 ==
  Enable : EnablePort  PropagateVarSize=During execution
  Counter Free-Running : simulink/Sources/Counter Free-Running  SystemSampleTime=-1  NumBits=32  tsamp=-1
  Out1 : Outport  InitialOutput=0
  wires:
  Counter Free-Running/1 -> Out1/1

== system stm32f4_rtc_lib/RTC Configure/Enabled Subsystem/Debouce3/Enabled Subsystem ==
  Enable : EnablePort  PropagateVarSize=During execution
  Counter Free-Running : simulink/Sources/Counter Free-Running  SystemSampleTime=-1  NumBits=32  tsamp=-1
  Out1 : Outport  InitialOutput=0
  wires:
  Counter Free-Running/1 -> Out1/1

== system stm32f4_rtc_lib/RTC Configure/Enabled Subsystem/Debouce3/Enabled Subsystem1 ==
  Enable : EnablePort  PropagateVarSize=During execution
  Bitwise Operator : simulink/Logic and Bit Operations/Bitwise Operator  logicop=AND  UseBitMask=on  BitMask=1  BitMaskRealWorld=Stored Integer
  Compare To Zero : simulink/Logic and Bit Operations/Compare To Zero  SystemSampleTime=-1  relop===  LogicOutDataTypeMode=uint8  ZeroCross=off
  Counter Free-Running : simulink/Sources/Counter Free-Running  SystemSampleTime=-1  NumBits=32  tsamp=-1
  Out1 : Outport  InitialOutput=0
  wires:
  Counter Free-Running/1 -> Bitwise Operator/1
  Bitwise Operator/1 -> Compare To Zero/1
  Compare To Zero/1 -> Out1/1

== system stm32f4_rtc_lib/RTC Configure/Enabled Subsystem/Debouce3/Enabled Subsystem4 ==
  Enable : EnablePort  PropagateVarSize=During execution
  Counter Free-Running : simulink/Sources/Counter Free-Running  SystemSampleTime=-1  NumBits=32  tsamp=-1
  Out1 : Outport  InitialOutput=0
  wires:
  Counter Free-Running/1 -> Out1/1

== system stm32f4_rtc_lib/RTC Configure/Enabled Subsystem/Debouce3/Enabled Subsystem5 ==
  Enable : EnablePort  PropagateVarSize=During execution
  Counter Free-Running : simulink/Sources/Counter Free-Running  SystemSampleTime=-1  NumBits=32  tsamp=-1
  Out1 : Outport  InitialOutput=0
  wires:
  Counter Free-Running/1 -> Out1/1

== system stm32f4_rtc_lib/RTC Configure/Enabled Subsystem/Generate Mode ID/Enabled Subsystem2 ==
  Enable : EnablePort  PropagateVarSize=During execution
  Bitwise Operator : simulink/Logic and Bit Operations/Bitwise Operator  logicop=AND  UseBitMask=on  BitMask=7  BitMaskRealWorld=Stored Integer
  Counter Free-Running : simulink/Sources/Counter Free-Running  SystemSampleTime=-1  NumBits=16  tsamp=-1
  Out1 : Outport  InitialOutput=0
  wires:
  Counter Free-Running/1 -> Bitwise Operator/1
  Bitwise Operator/1 -> Out1/1

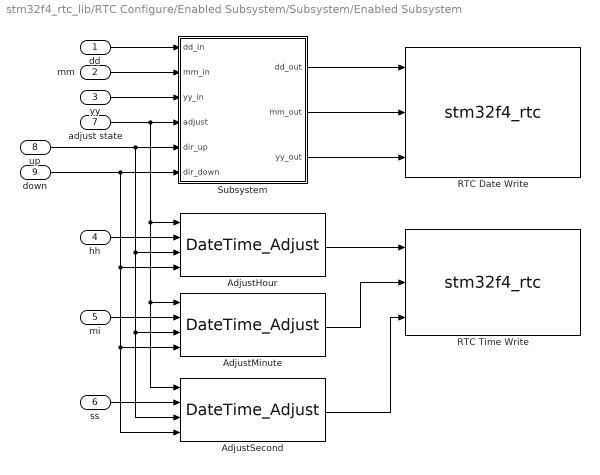
== system stm32f4_rtc_lib/RTC Configure/Enabled Subsystem/Subsystem/Enabled Subsystem ==
  dd : Inport
  mm : Inport  Port=2
  yy : Inport  Port=3
  hh : Inport  Port=4
  mi : Inport  Port=5
  ss : Inport  Port=6
  adjust state : Inport  Port=7
  up : Inport  Port=8
  down : Inport  Port=9
  AdjustHour : amg_high_precision_rtc/DateTime_Adjust  SystemSampleTime=-1  state=3  max=23  min=0
  AdjustMinute : amg_high_precision_rtc/DateTime_Adjust  SystemSampleTime=-1  state=4  max=59  min=0
  AdjustSecond : amg_high_precision_rtc/DateTime_Adjust  SystemSampleTime=-1  state=5  max=59  min=0
  RTC Date Write : S-Function  FunctionName=stm32f4_rtc  Parameters=inputtypearray,outputtypearray,confstr,sampletime,sampletimestr,blockid  SFunctionDeploymentMode=off  EnableBusSupport=off  mask(stm32f4_rtc){configuration=DateWrite, clocksource=LSE (32.768kHz), dataformat=BIN, hourformat=HourFormat_24, inputtypearray=[3 -1 -1 -1], outputtypearray=[0], confstr=["DateWrite","LSE (32.768kHz)","BIN","HourFormat_24"], sampletime=0.01, sampletimestr=0, blockid=stm32f4_rtc_libRTCConfigureEnabledSubsystemSubsystemEnabledSubsystemRTCDateWrite}
      mask prompts: clocksource "Clock source"; dataformat "Format"; hourformat "Hour format"; inputtypearray "Input type array"; outputtypearray "Output type array"; confstr "Configuration string"; sampletime "Sample time (sec)"; sampletimestr "Compiled sample time (sec) in string"
      mask init:
      | stm32f4_rtc_callback('init');
      mask Help: web(fullfile(waijungdocroot,'stm32f4_rtc_setup.htm'), '-browser')
      mask TypeOptions configuration: Setup | DateRead | TimeRead | DateWrite | TimeWrite
      mask Callback configuration: stm32f4_rtc_callback('configuration');
      mask TypeOptions clocksource: LSE (32.768kHz) | LSI
      mask TypeOptions dataformat: BCD | BIN
      mask Callback dataformat: stm32f4_rtc_callback('dataformat');
      mask TypeOptions hourformat: HourFormat_24 | HourFormat_12
      mask Callback confstr: stm32f4_rtc_callback('confstr');
      mask Callback sampletime: stm32f4_rtc_callback('sampletime');
      mask Callback sampletimestr: stm32f4_rtc_callback('sampletimestr');
      mask Callback blockid: stm32f4_rtc_callback('blockid');
      mask Display: text(0.95, 0.5, 'Module: RTC (DateWrite)\nFormat: BIN\nTs (sec): 0','ver','middle','hor','right');port_label('input', 1,'Date');port_label('input', 2,'Month');port_label('input', 3,'Year');
  RTC Time Write : S-Function  FunctionName=stm32f4_rtc  Parameters=inputtypearray,outputtypearray,confstr,sampletime,sampletimestr,blockid  SFunctionDeploymentMode=off  EnableBusSupport=off  mask(stm32f4_rtc){configuration=TimeWrite, clocksource=LSE (32.768kHz), dataformat=BIN, hourformat=HourFormat_24, inputtypearray=[3 -1 -1 -1], outputtypearray=[0], confstr=["TimeWrite","LSE (32.768kHz)","BIN","HourFormat_24"], sampletime=0.01, sampletimestr=0, blockid=stm32f4_rtc_libRTCConfigureEnabledSubsystemSubsystemEnabledSubsystemRTCTimeWrite}
      mask prompts: clocksource "Clock source"; dataformat "Format"; hourformat "Hour format"; inputtypearray "Input type array"; outputtypearray "Output type array"; confstr "Configuration string"; sampletime "Sample time (sec)"; sampletimestr "Compiled sample time (sec) in string"
      mask init:
      | stm32f4_rtc_callback('init');
      mask Help: web(fullfile(waijungdocroot,'stm32f4_rtc_setup.htm'), '-browser')
      mask TypeOptions configuration: Setup | DateRead | TimeRead | DateWrite | TimeWrite
      mask Callback configuration: stm32f4_rtc_callback('configuration');
      mask TypeOptions clocksource: LSE (32.768kHz) | LSI
      mask TypeOptions dataformat: BCD | BIN
      mask Callback dataformat: stm32f4_rtc_callback('dataformat');
      mask TypeOptions hourformat: HourFormat_24 | HourFormat_12
      mask Callback confstr: stm32f4_rtc_callback('confstr');
      mask Callback sampletime: stm32f4_rtc_callback('sampletime');
      mask Callback sampletimestr: stm32f4_rtc_callback('sampletimestr');
      mask Callback blockid: stm32f4_rtc_callback('blockid');
      mask Display: text(0.95, 0.5, 'Module: RTC (TimeWrite)\nFormat: BIN\nTs (sec): 0','ver','middle','hor','right');port_label('input', 1,'Hour');port_label('input', 2,'Minute');port_label('input', 3,'Second');
  Subsystem : Subsystem
  wires:
  dd/1 -> Subsystem/1(dd_in)
  mm/1 -> Subsystem/2(mm_in)
  yy/1 -> Subsystem/3(yy_in)
  adjust state/1 -> Subsystem/4(adjust), AdjustHour/1, AdjustMinute/1, AdjustSecond/1
  up/1 -> Subsystem/5(dir_up), AdjustHour/3, AdjustMinute/3, AdjustSecond/3
  down/1 -> Subsystem/6(dir_down), AdjustHour/4, AdjustMinute/4, AdjustSecond/4
  ss/1 -> AdjustSecond/2
  mi/1 -> AdjustMinute/2
  hh/1 -> AdjustHour/2
  AdjustHour/1 -> RTC Time Write/1
  AdjustSecond/1 -> RTC Time Write/3
  Subsystem/1(dd_out) -> RTC Date Write/1
  Subsystem/2(mm_out) -> RTC Date Write/2
  Subsystem/3(yy_out) -> RTC Date Write/3
  AdjustMinute/1 -> RTC Time Write/2

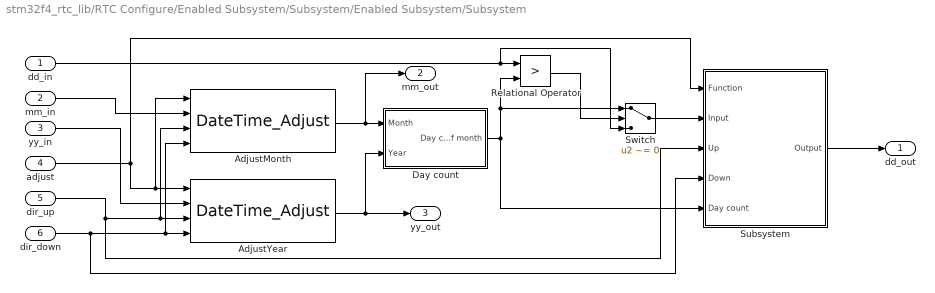
== system stm32f4_rtc_lib/RTC Configure/Enabled Subsystem/Subsystem/Enabled Subsystem/Subsystem ==
  dd_in : Inport
  mm_in : Inport  Port=2
  yy_in : Inport  Port=3
  adjust : Inport  Port=4
  dir_up : Inport  Port=5
  dir_down : Inport  Port=6
  AdjustMonth : amg_high_precision_rtc/DateTime_Adjust  SystemSampleTime=-1  state=1  max=12  min=1
  AdjustYear : amg_high_precision_rtc/DateTime_Adjust  SystemSampleTime=-1  state=2  max=99  min=0
  Day count : Subsystem
  Relational Operator : RelationalOperator  Operator=>  OutDataTypeStr=boolean
  Subsystem : Subsystem
  Switch : Switch  Criteria=u2 ~= 0
  dd_out : Outport
  mm_out : Outport  Port=2
  yy_out : Outport  Port=3
  wires:
  dir_down/1 -> AdjustYear/4, AdjustMonth/4, Subsystem/4(Down)
  dir_up/1 -> AdjustYear/3, AdjustMonth/3, Subsystem/3(Up)
  adjust/1 -> AdjustYear/1, AdjustMonth/1, Subsystem/1(Function)
  yy_in/1 -> AdjustYear/2
  mm_in/1 -> AdjustMonth/2
  AdjustYear/1 -> Day count/2(Year), yy_out/1
  AdjustMonth/1 -> Day count/1(Month), mm_out/1
  dd_in/1 -> Relational Operator/1, Switch/3
  Switch/1 -> Subsystem/2(Input)
  Day count/1(Day count of month) -> Relational Operator/2, Switch/1, Subsystem/5(Day count)
  Relational Operator/1 -> Switch/2
  Subsystem/1(Output) -> dd_out/1

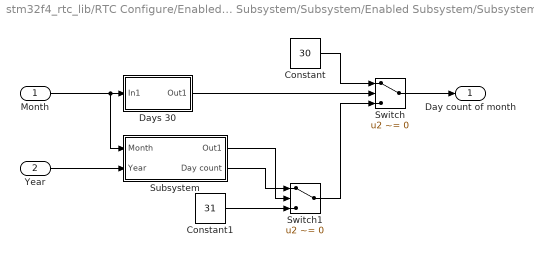
== system stm32f4_rtc_lib/RTC Configure/Enabled Subsystem/Subsystem/Enabled Subsystem/Subsystem/Day count ==
  Month : Inport
  Year : Inport  Port=2
  Constant : Constant  Value=30  OutDataTypeStr=uint8
  Constant1 : Constant  Value=31  OutDataTypeStr=uint8
  Days 30 : Subsystem
  Subsystem : Subsystem
  Switch : Switch  Criteria=u2 ~= 0
  Switch1 : Switch  Criteria=u2 ~= 0
  Day count of month : Outport
  wires:
  Days 30/1(Out1) -> Switch/2
  Constant/1 -> Switch/1
  Month/1 -> Days 30/1(In1), Subsystem/1(Month)
  Year/1 -> Subsystem/2(Year)
  Subsystem/1(Out1) -> Switch1/2
  Subsystem/2(Day count) -> Switch1/1
  Constant1/1 -> Switch1/3
  Switch1/1 -> Switch/3
  Switch/1 -> Day count of month/1

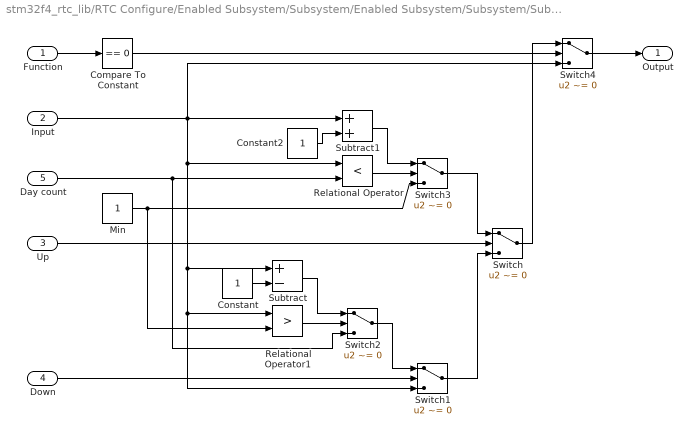
== system stm32f4_rtc_lib/RTC Configure/Enabled Subsystem/Subsystem/Enabled Subsystem/Subsystem/Subsystem ==
  Function : Inport
  Input : Inport  Port=2
  Up : Inport  Port=3
  Down : Inport  Port=4
  Day count : Inport  Port=5
  Compare To Constant : simulink/Logic and Bit Operations/Compare To Constant  SystemSampleTime=-1  relop===  const=0  LogicOutDataTypeMode=uint8  ZeroCross=off
  Constant : Constant  OutDataTypeStr=uint8
  Constant2 : Constant  OutDataTypeStr=uint8
  Min : Constant  OutDataTypeStr=uint8
  Relational Operator : RelationalOperator  Operator=<  OutDataTypeStr=boolean
  Relational Operator1 : RelationalOperator  Operator=>  OutDataTypeStr=boolean
  Subtract : Sum  Inputs=+-
  Subtract1 : Sum
  Switch{,1..4} (5 alike) : Switch  Criteria=u2 ~= 0
  Output : Outport
  wires:
  Switch1/1 -> Switch/3
  Input/1 -> Subtract/1, Switch1/3, Relational Operator1/1, Relational Operator/1, Subtract1/1, Switch4/3
  Relational Operator1/1 -> Switch2/2
  Subtract/1 -> Switch2/1
  Constant/1 -> Subtract/2
  Switch2/1 -> Switch1/1
  Relational Operator/1 -> Switch3/2
  Subtract1/1 -> Switch3/1
  Constant2/1 -> Subtract1/2
  Min/1 -> Switch3/3, Relational Operator1/2
  Day count/1 -> Relational Operator/2, Switch2/3
  Switch3/1 -> Switch/1
  Function/1 -> Compare To Constant/1
  Switch4/1 -> Output/1
  Compare To Constant/1 -> Switch4/2
  Switch/1 -> Switch4/1
  Down/1 -> Switch1/2
  Up/1 -> Switch/2

== system stm32f4_rtc_lib/RTC Configure/Enabled Subsystem/Subsystem/Enabled Subsystem/Subsystem/Day count/Days 30 ==
  In1 : Inport
  Bitwise Operator : simulink/Logic and Bit Operations/Bitwise Operator  logicop=OR  UseBitMask=off  NumInputPorts=4  BitMask=bin2dec('11011001')  BitMaskRealWorld=Stored Integer
  Compare To Constant : simulink/Logic and Bit Operations/Compare To Constant  SystemSampleTime=-1  relop===  const=6  LogicOutDataTypeMode=uint8  ZeroCross=off
  Compare To Constant1 : simulink/Logic and Bit Operations/Compare To Constant  SystemSampleTime=-1  relop===  const=4  LogicOutDataTypeMode=uint8  ZeroCross=off
  Compare To Constant2 : simulink/Logic and Bit Operations/Compare To Constant  SystemSampleTime=-1  relop===  const=9  LogicOutDataTypeMode=uint8  ZeroCross=off
  Compare To Constant3 : simulink/Logic and Bit Operations/Compare To Constant  SystemSampleTime=-1  relop===  const=11  LogicOutDataTypeMode=uint8  ZeroCross=off
  Out1 : Outport
  wires:
  Compare To Constant1/1 -> Bitwise Operator/1
  Compare To Constant/1 -> Bitwise Operator/2
  Compare To Constant2/1 -> Bitwise Operator/3
  Compare To Constant3/1 -> Bitwise Operator/4
  In1/1 -> Compare To Constant1/1, Compare To Constant/1, Compare To Constant2/1, Compare To Constant3/1
  Bitwise Operator/1 -> Out1/1

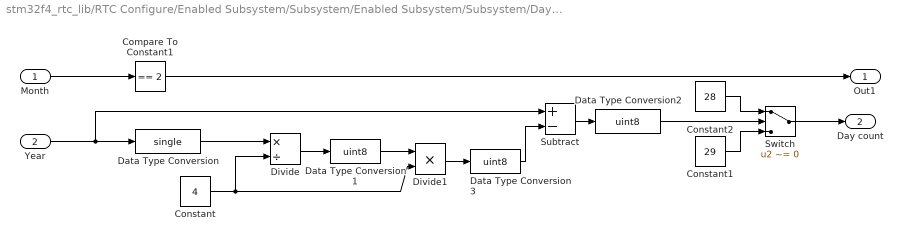
== system stm32f4_rtc_lib/RTC Configure/Enabled Subsystem/Subsystem/Enabled Subsystem/Subsystem/Day count/Subsystem ==
  Month : Inport
  Year : Inport  Port=2
  Compare To Constant1 : simulink/Logic and Bit Operations/Compare To Constant  SystemSampleTime=-1  relop===  const=2  LogicOutDataTypeMode=uint8  ZeroCross=off
  Constant : Constant  Value=4  OutDataTypeStr=single
  Constant1 : Constant  Value=29  OutDataTypeStr=uint8
  Constant2 : Constant  Value=28  OutDataTypeStr=uint8
  Data Type Conversion : DataTypeConversion  OutDataTypeStr=single
  Data Type Conversion1 : DataTypeConversion  OutDataTypeStr=uint8
  Data Type Conversion2 : DataTypeConversion  OutDataTypeStr=uint8
  Data Type Conversion3 : DataTypeConversion  OutDataTypeStr=uint8
  Divide : Product  Inputs=*/
  Divide1 : Product  Inputs=**
  Subtract : Sum  Inputs=+-
  Switch : Switch  Criteria=u2 ~= 0
  Out1 : Outport
  Day count : Outport  Port=2
  wires:
  Month/1 -> Compare To Constant1/1
  Compare To Constant1/1 -> Out1/1
  Year/1 -> Data Type Conversion/1, Subtract/1
  Data Type Conversion/1 -> Divide/1
  Constant/1 -> Divide/2, Divide1/2
  Divide/1 -> Data Type Conversion1/1
  Subtract/1 -> Data Type Conversion2/1
  Constant1/1 -> Switch/3
  Constant2/1 -> Switch/1
  Switch/1 -> Day count/1
  Data Type Conversion2/1 -> Switch/2
  Data Type Conversion1/1 -> Divide1/1
  Divide1/1 -> Data Type Conversion3/1
  Data Type Conversion3/1 -> Subtract/2
